simulink model "dvb_s2_channel_2"  (R2025b)
settings: Solver=VariableStepAuto  StartTime=0.0  StopTime=1  RelTol=1e-3
undefined symbols (not defined in the file or in its folder): pskmod, RRC_reseive, Ts
libraries: commsync2 x2, commdigbbndpm3 x2, commfilt2 x2, commchan3 x1, commrandsrc3 x1, dspsrcs4 x1, commrflib2 x1, simulink x1, dspsigops x1
settings Model: Creator=Пётр  LastModifiedBy=Пётр

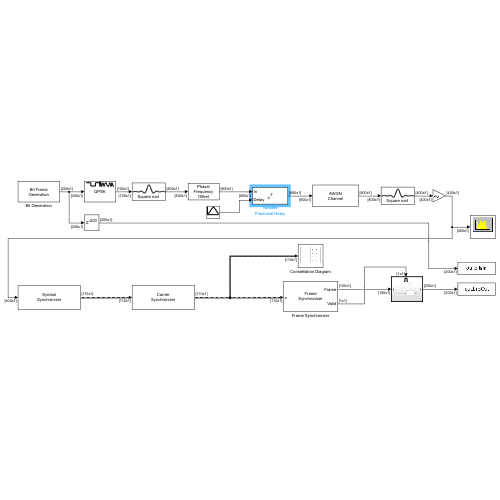
[thumbnail: Simulink's stored preview of the top-level diagram]
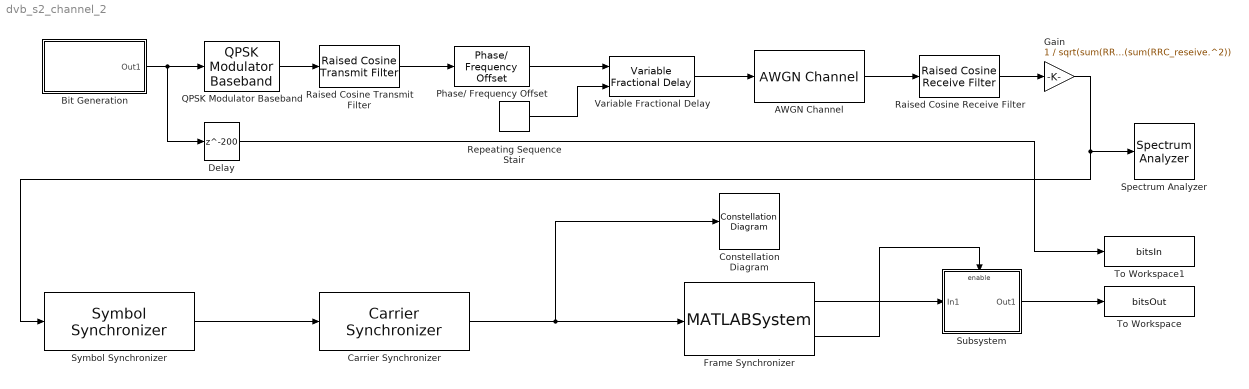
== system dvb_s2_channel_2 ==
  AWGN Channel : commchan3/AWGN Channel  LegacyMode=off  NoiseMethod="Signal to noise ratio  (SNR)"  noiseMode="Signal to noise ratio  (SNR)"  EbNo=10  EsNo=10  SNR=SNR  BitsPerSymbol=1  SignalPower=1  SpecifySymbolPeriod=off  SamplesPerSymbol=1  SymbolPeriod=1  VarianceSource=Parameter  Variance=1  RandomStream=Global stream  Seed=67  SimulateUsing=Code generation
  Bit Generation : Subsystem
      mask Display: disp('Bit Frame\nGeneration')
  Carrier Synchronizer : commsync2/Carrier Synchronizer  Modulation=QPSK  ModulationPhaseOffset=Auto  CustomPhaseOffset=0  SamplesPerSymbol=2  DampingFactor=0.707  NormalizedLoopBandwidth=0.05  EstimatedPhaseErrorOutputPort=off  SimulateUsing=Code generation
  Constellation Diagram : ConstellationDiagram  WindowPosition=[673.000000,246.000000,282.000000,294.000000,]  ScopeFrameLocation=window  SymbolsToDisplaySource=Property  SymbolsToDisplay=1000  ReferenceConstellation="[0.70711+0.70711i        -0.70711+0.70711i        -0.70711-0.70711i         0.70711-0.70711i]"  ShowLegend=on  MeasurementInterval=1000
  Delay : Delay  DelayLength=200  InputProcessing=Columns as channels (frame based)  UseCircularBuffer=on
  Frame Synchronizer : MATLABSystem  System=FrameSynchronizer  Preamble=pskmod([1 0 0 1 0 1 1 0 1 1 1 0 1 0 1 1 0 1 1 0 1 0 0 1 0 1 1 0 1 1 1 0 1 0 1 1 0 1 1 0]',4,pi/4,'InputType','bit')  Threshold=15  OutputLength=100  SimulateUsing=Code generation
      mask Type: FrameSynchronizer
  Gain : Gain  Gain="1 / sqrt(sum(RRC_reseive.^2)) /  sqrt(sum(RRC_reseive.^2))"
  Phase/ Frequency Offset : commrflib2/Phase// Frequency Offset  phaseOffset=0  freqPort=off  freqOffset=2000
  QPSK Modulator Baseband : commdigbbndpm3/QPSK Modulator Baseband  InType=Bit  Enc=Gray  Ph=pi/4  outDtype=double  outWordLen=16  outUDDataType=sfix(16)  outFracLenMode=Best precision  outFracLen=15  outDataTypeStr=double  outLastDataTypeStr=double
  Raised Cosine Receive Filter : commfilt2/Raised Cosine Receive Filter  filtType=Square root  R=0.25  filtSpan=10  N=8  downFactor=2  downOffset=0  filterGain=10  InputProcessing=Columns as channels (frame based)  RateOptions=Enforce single-rate processing  framing=Mute  checkCoeff=on  variableName=RRC_reseive  currentFiltSpan=10  D=5  inputOffset=0  sampMode=Mute  saveAsFlag=0  rateMode=Downsampling  checkGain=Normalized  launchFVT=on  roundingMode=Floor  overflowMode=off  coeffDataTypeStr=Inherit: Same word length as input  coeffMin=[]  coeffMax=[]  coeffLastDataTypeStr=Inherit: Same word length as input  accumDataTypeStr=Inherit: Same as product output  accumLastDataTypeStr=Inherit: Same as product output  outputDataTypeStr=Inherit: Same as accumulator  outputMin=[]  outputMax=[]  outputLastDataTypeStr=Inherit: Same as accumulator
  Raised Cosine Transmit Filter : commfilt2/Raised Cosine Transmit Filter  filtType=Square root  R=0.25  filtSpan=10  N=8  filterGain=10  InputProcessing=Columns as channels (frame based)  RateOptions=Enforce single-rate processing  framing=Mute  checkCoeff=off  variableName=rcTxFilt  checkGain=Normalized  sampMode=Mute  saveAsFlag=0  currentFiltSpan=10  D=(10)/2  launchFVT=on  roundingMode=Floor  overflowMode=off  coeffDataTypeStr=Inherit: Same word length as input  coeffMin=[]  coeffMax=[]  coeffLastDataTypeStr=Inherit: Same word length as input  outputDataTypeStr=Inherit: Same as accumulator  outputMin=[]  outputMax=[]  outputLastDataTypeStr=Inherit: Same as accumulator
  Repeating Sequence Stair : simulink/Sources/Repeating Sequence Stair  OutValues=[0:0.1:0.9 0.8:-0.1:0.1]  tsamp=-1  OutMin=[]  OutMax=[]  OutDataTypeStr=double  OutputDataTypeScalingMode=double  OutDataType=fixdt(0,8)  ConRadixGroup=Best Precision: Vector-wise  OutScaling=2^-12
  Spectrum Analyzer : SpectrumAnalyzer  WindowPosition=[42.000000,231.000000,567.000000,316.000000,]  ScopeFrameLocation=window  SampleRate=100000000  Span=1000000  StartFrequency=-500000  StopFrequency=500000  AveragingMethod=Exponential  YLimits=[-99.3045 24.9076]  ShowLegend=on  AllowFFTLengthLessThanSamplesPerUpdate=on
  Subsystem : Subsystem
  Symbol Synchronizer : commsync2/Symbol Synchronizer  Modulation=PAM/PSK/QAM  TimingErrorDetector=Gardner (non-data-aided)  SamplesPerSymbol=4  DampingFactor=1  NormalizedLoopBandwidth=0.01  DetectorGain=2.7  TimingErrorOutputPort=off  SimulateUsing=Code generation
  To Workspace : ToWorkspace  VariableName=bitsOut  SampleTime=-1
      settings: Save2DSignal=2-D array (concatenate along first dimension)
  To Workspace1 : ToWorkspace  VariableName=bitsIn  SampleTime=-1
      settings: Save2DSignal=2-D array (concatenate along first dimension)
  Variable Fractional Delay : dspsigops/Variable Fractional Delay  mode=OBSOLETE  modeActive=Linear  L=4  FarrowL=4  R=10  alpha=1  dmax=400  InputProcessing=Columns as channels (frame based)  ic=0  noDFT=off  fallbackFIR=Clip to the minimum value necessary for centered kernel  fallbackFarrow=Clip to the minimum value necessary for centered kernel  roundingMode=Zero  overflowMode=off
  wires:
  AWGN Channel/1 -> Raised Cosine Receive Filter/1
  Gain/1 -> Spectrum Analyzer/1, Symbol Synchronizer/1
  Raised Cosine Receive Filter/1 -> Gain/1
  QPSK Modulator Baseband/1 -> Raised Cosine Transmit Filter/1
  Symbol Synchronizer/1 -> Carrier Synchronizer/1
  Repeating Sequence Stair/1 -> Variable Fractional Delay/2
  Bit Generation/1(Out1) -> Delay/1, QPSK Modulator Baseband/1
  Frame Synchronizer/1 -> Subsystem/1(In1)
  Subsystem/1(Out1) -> To Workspace/1
  Delay/1 -> To Workspace1/1
  Raised Cosine Transmit Filter/1 -> Phase/ Frequency Offset/1
  Variable Fractional Delay/1 -> AWGN Channel/1
  Frame Synchronizer/2 -> Subsystem/Enable
  Phase/ Frequency Offset/1 -> Variable Fractional Delay/1
  Carrier Synchronizer/1 -> Constellation Diagram/1, Frame Synchronizer/1

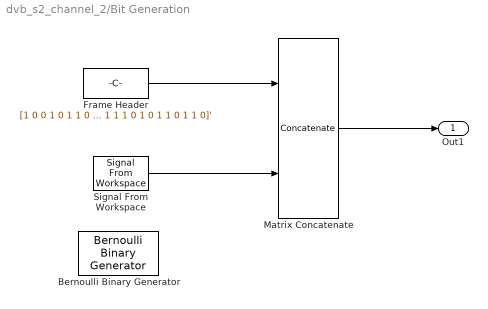
== system dvb_s2_channel_2/Bit Generation ==
  Bernoulli Binary Generator : commrandsrc3/Bernoulli Binary Generator  ProbabilityOfZero=0.5  SeedSource=Parameter  Seed=61  SampleTime=1  SamplesPerFrame=160  OutputDataType=double  SimulateUsing=Interpreted execution
  Frame Header : Constant  Value=[1 0 0 1 0 1 1 0 1 1 1 0 1 0 1 1 0 1 1 0 1 0 0 1 0 1 1 0 1 1 1 0 1 0 1 1 0 1 1 0]'  VectorParams1D=off  OutDataTypeStr=double
  Matrix Concatenate : Concatenate  Mode=Multidimensional array
  Signal From Workspace : dspsrcs4/Signal From Workspace  X=bitsIn  Ts=Ts  nsamps=160  OutputAfterFinalValue=Setting to zero  ignoreOrWarnInputAndFrameLengths=off  OutputFrames=off
  Out1 : Outport  VectorParamsAs1DForOutWhenUnconnected=off
  wires:
  Matrix Concatenate/1 -> Out1/1
  Frame Header/1 -> Matrix Concatenate/1
  Signal From Workspace/1 -> Matrix Concatenate/2

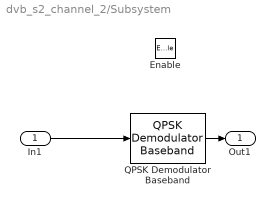
== system dvb_s2_channel_2/Subsystem ==
  In1 : Inport
  Enable : EnablePort
  QPSK Demodulator Baseband : commdigbbndpm3/QPSK Demodulator Baseband  OutType=Bit  DecType=Hard decision  VarSource=Dialog  Variance=1  Dec=Gray  Ph=pi/4  outDtype1=Inherit via internal rule  outDtype2=Inherit via internal rule  derotateFactorWordLen=16  derotateFactorDataTypeStr=Inherit: Same word length as input  derotateFactorLastDataTypeStr=Inherit: Same word length as input
      settings: LibrarySourceBlock=|
      | commhdldigbbndpm/QPSK
      | Demodulator
      | Baseband
  Out1 : Outport
  wires:
  In1/1 -> QPSK Demodulator Baseband/1
  QPSK Demodulator Baseband/1 -> Out1/1
